simulink model "EXP1_EX14"  (R2021b)
settings: Solver=VariableStepAuto  StartTime=0.0  StopTime=20.0  RelTol=1e-3
values from neighbouring files (symbols this model uses):
  a = 0.1    [EXP1.m]
  GainDx = (1-exp(-Tx))/(1-exp(-0.1*Tx))    [EXP1.m]
  p1 = exp(-Tx)    [EXP1.m]
  z1 = exp(-0.1*Tx)    [EXP1.m]
settings Model: Creator=luang  LastModifiedBy=luang

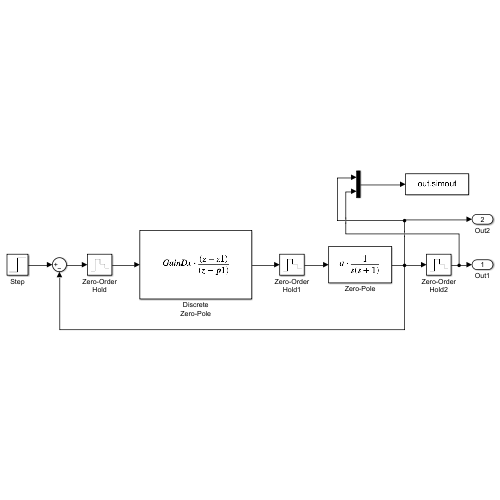
[thumbnail: Simulink's stored preview of the top-level diagram]
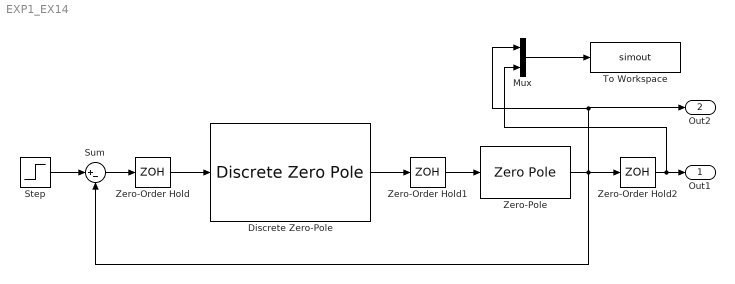
== system EXP1_EX14 ==
  Discrete Zero-Pole : DiscreteZeroPole  Zeros=[z1]  Poles=[p1]  Gain=GainDx  SampleTime=-1
  Mux : Mux  Inputs=2
  Step : Step  SampleTime=0
  Sum : Sum  Inputs=|+-
  To Workspace : ToWorkspace  VariableName=simout  SaveFormat=Structure With Time  SampleTime=-1
  Zero-Order Hold : ZeroOrderHold  SampleTime=-1
  Zero-Order Hold1 : ZeroOrderHold  SampleTime=-1
  Zero-Order Hold2 : ZeroOrderHold  SampleTime=-1
  Zero-Pole : ZeroPole  Zeros=[]  Poles=[0 -1]  Gain=a
  Out1 : Outport
  Out2 : Outport  Port=2
  wires:
  Step/1 -> Sum/1
  Sum/1 -> Zero-Order Hold/1
  Zero-Order Hold/1 -> Discrete Zero-Pole/1
  Discrete Zero-Pole/1 -> Zero-Order Hold1/1
  Zero-Order Hold1/1 -> Zero-Pole/1
  Zero-Pole/1 -> Mux/1, Out2/1, Zero-Order Hold2/1, Sum/2
  Zero-Order Hold2/1 -> Mux/2, Out1/1
  Mux/1 -> To Workspace/1
